simulink model "Sim_base"  (R2018b)
settings: Solver=VariableStepAuto  StartTime=0.0  StopTime=22  RelTol=1e-3
values from neighbouring files (symbols this model uses):
  q_0 = zeros(5,1).'    [DATAsim.m]
undefined symbols (not defined in the file or in its folder): limit_check, v_max
libraries: simulink x1
settings Model: Creator=Francesco Gennari  LastModifiedBy=RaffaelePC

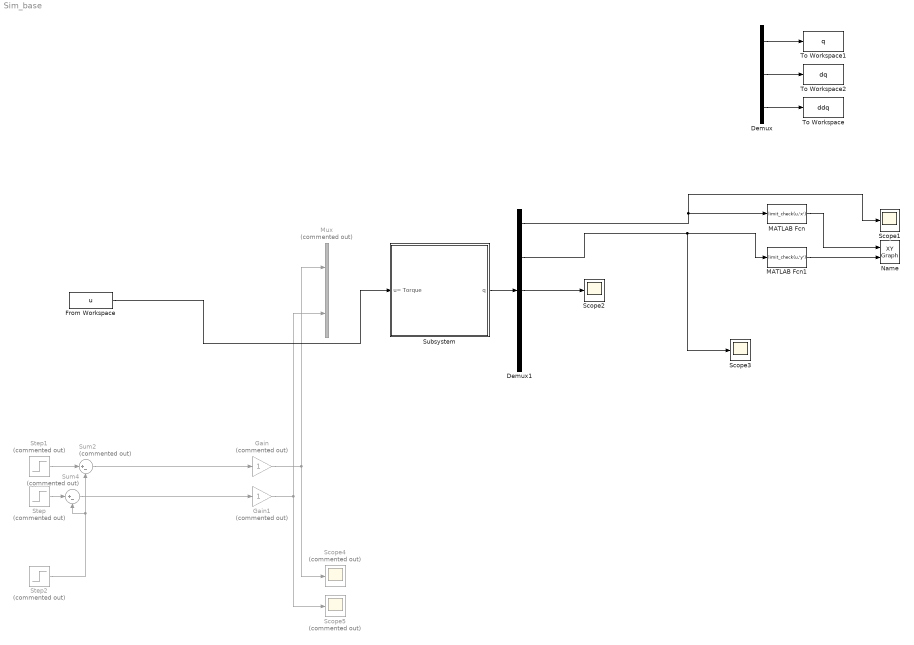
== system Sim_base ==
  Demux : Demux  Outputs=3
  Demux1 : Demux  Outputs=[1 1 1 1 1]
  From Workspace : FromWorkspace  VariableName=u  SampleTime=0
  Gain : Gain  Commented=on
  Gain1 : Gain  Commented=on
  MATLAB Fcn : MATLABFcn  MATLABFcn=limit_check(u,'x')
  MATLAB Fcn1 : MATLABFcn  MATLABFcn=limit_check(u,'y')
  Mux : Mux  Commented=on  Inputs=2
  Name : simulink/Sinks/XY Graph  xmin=-5  xmax=5  ymin=-5  ymax=5  st=-1
  Scope1 : Scope
  Scope2 : Scope
  Scope3 : Scope
  Scope4 : Scope  Commented=on
  Scope5 : Scope  Commented=on
  Step : Step  Commented=on  After=4  SampleTime=0
  Step1 : Step  Commented=on  After=4  SampleTime=0
  Step2 : Step  Commented=on  Time=2  After=4  SampleTime=0
  Subsystem : Subsystem
  Sum2 : Sum  Commented=on  Inputs=|+-
  Sum4 : Sum  Commented=on  Inputs=|+-
  To Workspace : ToWorkspace  VariableName=ddq  SaveFormat=Timeseries  SampleTime=-1
  To Workspace1 : ToWorkspace  VariableName=q  SaveFormat=Timeseries  SampleTime=-1
  To Workspace2 : ToWorkspace  VariableName=dq  SaveFormat=Timeseries  SampleTime=-1
  wires:
  Demux/2 -> To Workspace2/1
  Demux/1 -> To Workspace1/1
  Demux/3 -> To Workspace/1
  Subsystem/1(q) -> Demux1/1
  Demux1/1 -> MATLAB Fcn/1, Scope1/1
  Demux1/2 -> MATLAB Fcn1/1, Scope3/1
  Sum2/1 -> Gain/1
  Sum4/1 -> Gain1/1
  Gain/1 -> Scope4/1, Mux/1
  Gain1/1 -> Scope5/1, Mux/2
  Demux1/3 -> Scope2/1
  MATLAB Fcn1/1 -> Name/2
  MATLAB Fcn/1 -> Name/1
  Step2/1 -> Sum4/2, Sum2/2
  Step1/1 -> Sum2/1
  Step/1 -> Sum4/1
  From Workspace/1 -> Subsystem/1(u= Torque)

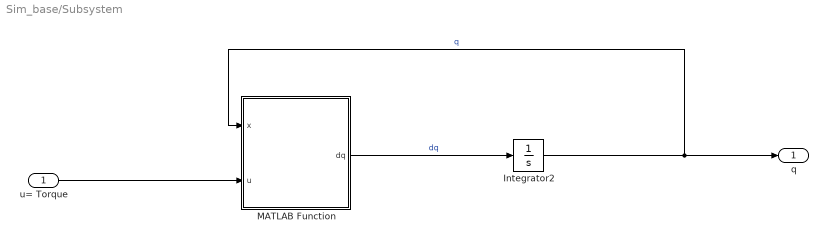
== system Sim_base/Subsystem ==
  u= Torque : Inport
  Integrator2 : Integrator  InitialCondition=q_0  UpperSaturationLimit=v_max  LowerSaturationLimit=-v_max  ContinuousStateAttributes='velocity'
  MATLAB Function : MATLAB Function  TreatAsAtomicUnit=on
  q : Outport
  wires:
  Integrator2/1 -> q/1, MATLAB Function/1(x)  "q"
  MATLAB Function/1(dq) -> Integrator2/1  "dq"
  u= Torque/1 -> MATLAB Function/2(u)

== matlab function Sim_base/Subsystem/MATLAB Function ==
  data: x input; dq output; u input
function dq   = sys_dynamics(x,u)

[A,F,D] = matriceseval(x);
 
dq=A*x+F*u+D;


end
